simulink model "dyskretny_i_ciagly"  (R2023a)
settings: Solver=VariableStepAuto  StartTime=0.0  StopTime=200  RelTol=1e-3
values from neighbouring files (symbols this model uses):
  a0 = 0.000531632    [zad1.m]    (also in zad2_8.m; zadanie_dodatkowe.m)
  a1 = 0.0207337    [zad1.m]    (also in zad2_8.m; zadanie_dodatkowe.m)
  a2 = 0.254652    [zad1.m]    (also in zad2_8.m; zadanie_dodatkowe.m)
  alpha1 = -0.3    [zad1.m]    (also in zad2_8.m; zadanie_dodatkowe.m)
  alpha2 = -0.55    [zad1.m]    (also in zad2_8.m; zadanie_dodatkowe.m)
  alpha3 = 0.4    [zad1.m]    (also in zad2_8.m; zadanie_dodatkowe.m)
  alpha4 = 0.21    [zad1.m]    (also in zad2_8.m; zadanie_dodatkowe.m)
  b0 = 0.00122807    [zad1.m]    (also in zad2_8.m; zadanie_dodatkowe.m)
  T = 5    [zad2_8.m]
undefined symbols (not defined in the file or in its folder): DiscIntNeverNeededParam
settings Model: Creator=adams  LastModifiedBy=adams

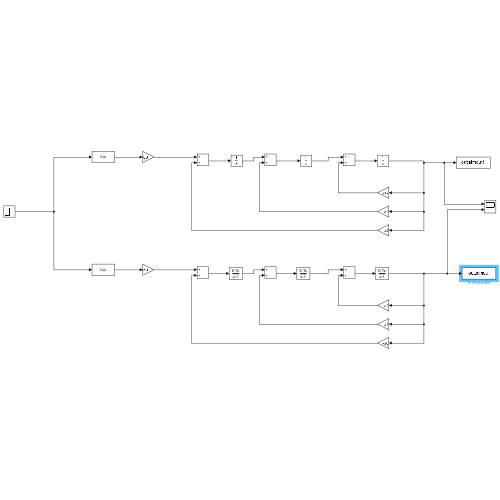
[thumbnail: Simulink's stored preview of the top-level diagram]
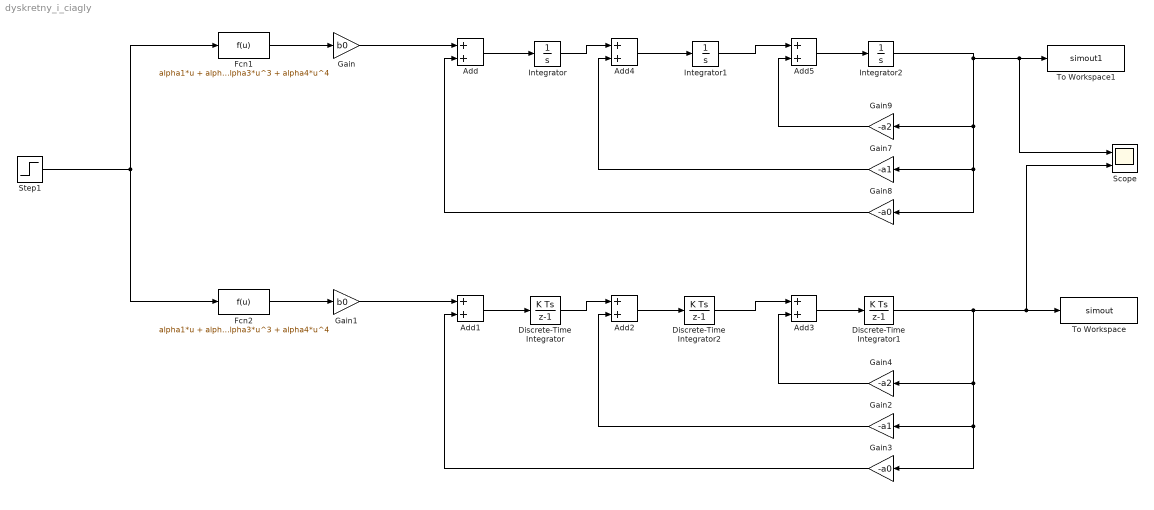
== system dyskretny_i_ciagly ==
  Add{,1..5} (6 alike) : Sum
  Discrete-Time Integrator : DiscreteIntegrator  SampleTime=T  ICPrevOutput=DiscIntNeverNeededParam  ICPrevScaledInput=DiscIntNeverNeededParam
  Discrete-Time Integrator1 : DiscreteIntegrator  SampleTime=T  ICPrevOutput=DiscIntNeverNeededParam  ICPrevScaledInput=DiscIntNeverNeededParam
  Discrete-Time Integrator2 : DiscreteIntegrator  SampleTime=T  ICPrevOutput=DiscIntNeverNeededParam  ICPrevScaledInput=DiscIntNeverNeededParam
  Fcn1 : Fcn  Expr=alpha1*u + alpha2*u^2 + alpha3*u^3 + alpha4*u^4
  Fcn2 : Fcn  Expr=alpha1*u + alpha2*u^2 + alpha3*u^3 + alpha4*u^4
  Gain : Gain  Gain=b0
  Gain1 : Gain  Gain=b0
  Gain2 : Gain  Gain=-a1
  Gain3 : Gain  Gain=-a0
  Gain4 : Gain  Gain=-a2
  Gain7 : Gain  Gain=-a1
  Gain8 : Gain  Gain=-a0
  Gain9 : Gain  Gain=-a2
  Integrator : Integrator
  Integrator1 : Integrator
  Integrator2 : Integrator
  Scope : Scope  NumInputPorts=2
  Step1 : Step  SampleTime=0
  To Workspace : ToWorkspace  VariableName=simout  SaveFormat=Structure With Time  SampleTime=0.001
  To Workspace1 : ToWorkspace  VariableName=simout1  SaveFormat=Structure With Time  SampleTime=-1
  wires:
  Integrator1/1 -> Add5/1
  Integrator2/1 -> Scope/1, To Workspace1/1, Gain7/1, Gain8/1, Gain9/1
  Gain9/1 -> Add5/2
  Add5/1 -> Integrator2/1
  Add/1 -> Integrator/1
  Gain8/1 -> Add/2
  Gain7/1 -> Add4/2
  Integrator/1 -> Add4/1
  Gain/1 -> Add/1
  Add4/1 -> Integrator1/1
  Fcn1/1 -> Gain/1
  Fcn2/1 -> Gain1/1
  Add2/1 -> Discrete-Time Integrator2/1
  Add1/1 -> Discrete-Time Integrator/1
  Add3/1 -> Discrete-Time Integrator1/1
  Step1/1 -> Fcn1/1, Fcn2/1
  Discrete-Time Integrator1/1 -> Scope/2, To Workspace/1, Gain2/1, Gain3/1, Gain4/1
  Discrete-Time Integrator2/1 -> Add3/1
  Gain4/1 -> Add3/2
  Discrete-Time Integrator/1 -> Add2/1
  Gain3/1 -> Add1/2
  Gain1/1 -> Add1/1
  Gain2/1 -> Add2/2
